simulink model "Jakub_Baczyk_1_Projekt_2_Ukl_c"  (R2015a)
settings: Solver=ode45  StartTime=0.0  StopTime=25  RelTol=1e-3
undefined symbols (not defined in the file): b1
settings Model: Creator=238  LastModifiedBy=lenovo

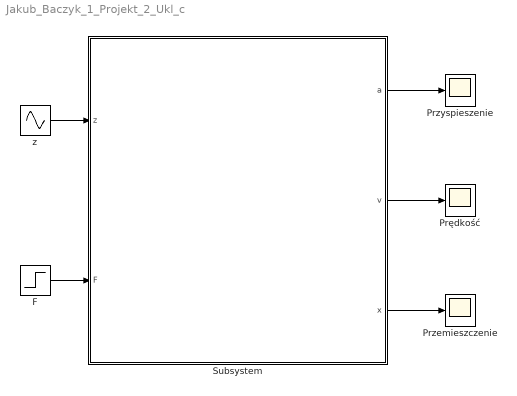
== system Jakub_Baczyk_1_Projekt_2_Ukl_c ==
  F : Step  Time=0  SampleTime=0
  Przemieszczenie : Scope
  Przyspieszenie : Scope
  Prędkość : Scope
      settings: SaveName=ScopeData2
  Subsystem : Subsystem  mask(Układ masa sprężyna tłumik){m=10, v0=0, x0=0, c2=3, c1=5, bb1=3}
      mask prompts: m "Masa [kg]"; v0 "Prędkość początkowa [m/s]"; x0 "Przemieszczenie początkowe [m]"; c2 "Sztywnosc sprezyny c1[]"; c1 "Sztywność sprężyny c2[]"; bb1 "Wspolczynnik tlumienia b1[]"
      mask help:
      | Zmodelowany układ mechaniczny, który opiera się na tłumiku b1 i sprężynach
      | c1 oraz c2. Na klocek działają wymuszenie siłowe (F) oraz kinematyczne (z).
      | Przemieszczenie zostało określone jako "x". Poniżej można wprowadzić
      | parametry pozwalające śledzić charakterystykę zachowania się układu.
      mask Help:
      | <html>
      | <img src="C:\Users\lenovo\Desktop\c.png">
      | <p> Sygnały wejściowe modelu to:
      | F- wymuszenie siłowe
      | z- wymuszenie kinematyczne
      | </p>
      | <p> Parametry układu:
      | m- masa klocka
      | v0-prędkość początkowa klocka,
      | x0-przemieszczenie początkowe klocka,
      | b1- wartość tłumienia poszczególnych tłumików,
      | c1,c2- wartość sztywności poszczególnych sprężyn
      | </p>
      | <p> Przebiegi, które możemy rejestrować:
      | x- przemieszczenie się klocka,
      | V- prędkość klocka,
      | a- przyspieszenie klocka
      | </p>
      | Aby zobaczyć przebieg charakterystyki należy kliknąć na odpowiedni wyświetlacz.
      | <p>
      | Uwagi!
      | - wpisywana masa musi być dodatnia
      | -należy podać wszystkie parametry w celu odzwierciedlenia przebiegu
      | </html>
      mask Callback m:
      | if str2num(get_param(gcb,'m'))<=0
      |     error('masa musi być dodatnia')
      | end
      mask TypeOptions bb1: 1 | 2 | 3 | 4 | 5 | 6 | 7 | 8 | 9 | 10
      mask Callback bb1: b1=str2num(get_param(gcb,'bb1'));
      mask Display:
      | color('blue')% kolor lini
      | %kreski pod linią
      | plot([0.12 0.09],[0.1 0.05])
      | plot([0.15 0.12],[0.1 0.05])
      | plot([0.18 0.15],[0.1 0.05])
      | plot([0.21 0.18],[0.1 0.05])
      | plot([0.24 0.21],[0.1 0.05])
      | plot([0.27 0.24],[0.1 0.05])
      | plot([0.30 0.27],[0.1 0.05])
      | plot([0.33 0.3],[0.1 0.05])
      | plot([0.36 0.33],[0.1 0.05])
      | plot([0.39 0.36],[0.1 0.05])
      | plot([0.42 0.39],[0.1 0.05])
      | plot([0.45 0.42,],[0.1 0.05])
      | plot([0.48 0.45],[0.1 0.05])
      | plot([0.51 0.48],[0.1 0.05])
      | plot([0.54 0.51],[0.1 0.05])
      | plot([0.57 0.54],[0.1 0.05])
      | plot([0.6 0.57],[0.1 0.05])
      | plot([0.63 0.6],[0.1 0.05])
      | plot([0.66 0.63],[0.1 0.05])
      | plot([0.69 0.66],[0.1 0.05])
      | plot([0.72 0.69],[0.1 0.05])
      | plot([0.75 0.72],[0.1 0.05])
      | plot([0.78 0.75],[0.1 0.05])
      | plot([0.81 0.78],[0.1 0.05])
      | plot([0.84 0.81],[0.1 0.05])
      | plot([0.87 0.84],[0.1 0.05])
      | 
      | plot([0.1 0.9],[0.1 0.1]) %współrzędne x i y, pierwsza linia pozioma
      | plot([0.1 0.9],[0.103 0.103]) %pogrubienie linii
      | plot([0.4 0.4],[0.1 0.2]) %pod tłumikem
      | %tłumik b1
      | plot([0.35 0.45],[0.2 0.2])
      | plot([0.35 0.35],[0.2 0.23])
      | plot([0.45 0.45],[0.2 0.23])
      | plot([0.36 0.44],[0.23 0.23])
      | plot([0.4 0.4],[0.23 0.38]) %nad tłumikiem
      | plot([0.7 0.7],[0.1 0.15]) %pod spręzyną
      | %sprężyna c2
      | plot([0.7 0.65],[0.15 0.16])
      | plot([0.65 0.75],[0.16 0.17])
      | plot([0.75 0.65],[0.17 0.185])
      | plot([0.75 0.65],[0.17 0.185])
      | plot([0.65 0.75],[0.185 0.2])
      | plot([0.75 0.7],[0.2 0.21])
      | plot([0.7 0.7],[0.21 0.27]) %nad sprężyną c2
      | %sprężyna c1
      | plot([0.7 0.65],[0.27 0.28])
      | plot([0.65 0.75],[0.28 0.29])
      | plot([0.75 0.65],[0.29 0.305])
      | plot([0.75 0.65],[0.29 0.305])
      | plot([0.65 0.75],[0.305 0.32])
      | plot([0.75 0.7],[0.32 0.33])
      | plot([0.7 0.7],[0.33 0.38])%nad sprężyną c1
      | %masa
      | plot([0.3 0.8],[0.38 0.38])
      | plot([0.3 0.8],[0.68 0.68])
      | plot([0.3 0.3],[0.38 0.68])
      | plot([0.8 0.8],[0.38 0.68])
      | %strzałka dla x
      | plot([0.3 0.15],[0.6 0.6])
      | plot([0.18 0.18],[0.6 0.52])
      | %strzałka dla z
      | plot([0.445 0.445],[0.8 0.68])
      | %strzałka dla F
      | plot([0.65 0.65],[0.8 0.68])
      | patch([0.178 0.189 0.2],[0.53 0.495 0.53],[0 0 1])%grot dla x
      | patch([0.43 0.45 0.47],[0.71 0.675 0.71],[0 0 1])%grot dla z
      | patch([0.63 0.65 0.67],[0.71 0.675 0.71],[0 0 1])%grot dla F
      | color('black')
      | %opis parametrów
      | text(0.55,0.55,'m')
      | text(0.45,0.28,'b1')
      | text(0.75,0.23,'c2')
      | text(0.75,0.35,'c1')
      | text(0.21,0.55,'x')
      | text(0.45,0.85,'z')
      | text(0.65,0.85,'F')
      | %opis wejść/wyjść
      | port_label('output', 1, 'a')
      | port_label('output', 2, 'v')
      | port_label('output', 3, 'x')
      | port_label('input', 1, 'z')
      | port_label('input', 2, 'F')
  z : Sin  Amplitude=0  Frequency=0  SampleTime=0
  wires:
  z/1 -> Subsystem/1(z)
  F/1 -> Subsystem/2(F)
  Subsystem/1(a) -> Przyspieszenie/1
  Subsystem/2(v) -> Prędkość/1
  Subsystem/3(x) -> Przemieszczenie/1

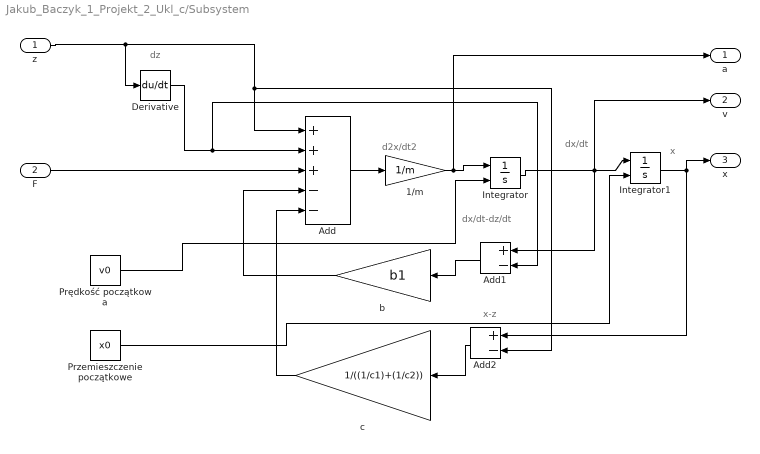
== system Jakub_Baczyk_1_Projekt_2_Ukl_c/Subsystem ==
  note: x-z
  note: dx/dt-dz/dt
  note: x
  note: dx/dt
  note: d2x/dt2
  note: dz
  z : Inport
  F : Inport  Port=2
  1/m : Gain  Gain=1/m
  Add : Sum  Inputs=+++--
  Add1 : Sum  Inputs=+-
  Add2 : Sum  Inputs=+-
  Derivative : Derivative
  Integrator : Integrator  InitialConditionSource=external
  Integrator1 : Integrator  InitialConditionSource=external
  Przemieszczenie początkowe : Constant  Value=x0
  Prędkość początkowa : Constant  Value=v0
  b : Gain  Gain=b1
  c : Gain  Gain=1/((1/c1)+(1/c2))
  a : Outport
  v : Outport  Port=2
  x : Outport  Port=3
  wires:
  Add2/1 -> c/1
  c/1 -> Add/5
  z/1 -> Derivative/1, Add2/2, Add/1
  F/1 -> Add/3
  Integrator1/1 -> x/1, Add2/1
  1/m/1 -> a/1, Integrator/1
  Przemieszczenie początkowe/1 -> Integrator1/2
  Prędkość początkowa/1 -> Integrator/2
  Derivative/1 -> Add1/2, Add/2
  Add1/1 -> b/1
  Add/1 -> 1/m/1
  b/1 -> Add/4
  Integrator/1 -> v/1, Add1/1, Integrator1/1
